simulink model "Multilink_Robot_Arm_control"  (R2019b)
settings: Solver=VariableStepAuto  StartTime=0.0  StopTime=10.0  RelTol=1e-3
libraries: fl_lib x64, fl_ps_legacy_lib x32, nesl_utility x16, simulink x8, ee_lib x8, simulink_extras x4
(part 1 of 2)
settings Model: Creator=Shivanshu  LastModifiedBy=Shivanshu
settings DebuggingCC: SFMachineParentedDataDiag=error

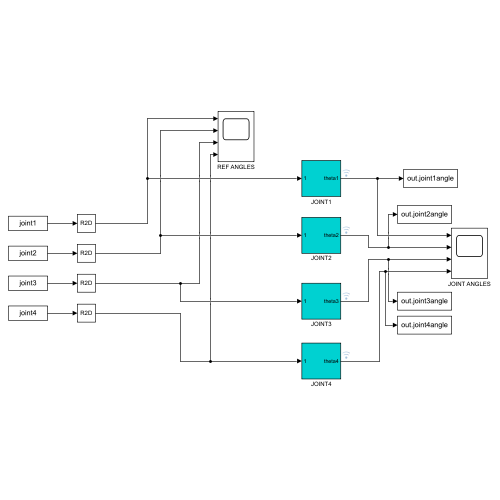
[thumbnail: Simulink's stored preview of the top-level diagram]
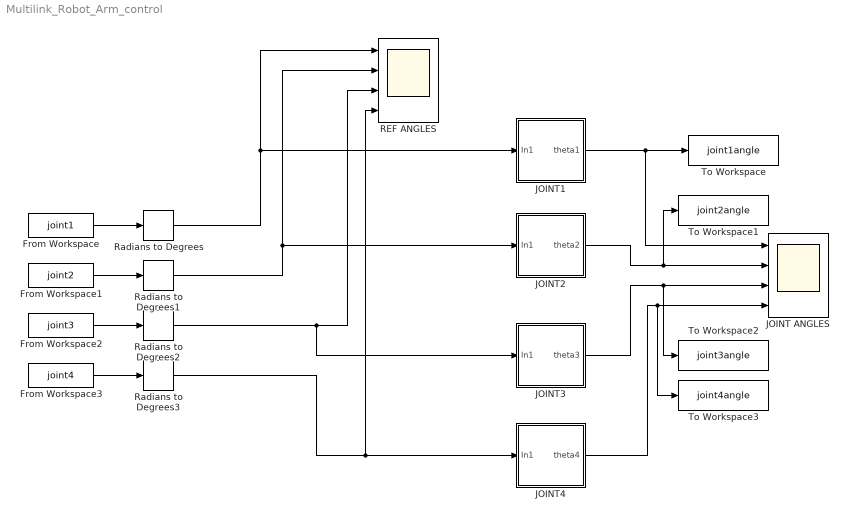
== system Multilink_Robot_Arm_control ==
  From Workspace : FromWorkspace  VariableName=joint1
  From Workspace1 : FromWorkspace  VariableName=joint2
  From Workspace2 : FromWorkspace  VariableName=joint3
  From Workspace3 : FromWorkspace  VariableName=joint4
  JOINT ANGLES : Scope  NumInputPorts=4
  JOINT1 : Subsystem  RequirementInfo={} %GIDa_a5111363_163f_4345_b806_ea7696c3bbc6
  JOINT2 : Subsystem  RequirementInfo={} %GIDa_53c2f0f4_4c39_4c98_aaeb_3fe1813d08cd
  JOINT3 : Subsystem  RequirementInfo={} %GIDa_0e8d513e_7ac6_45e5_95f2_a8ebfc01a2ff
  JOINT4 : Subsystem  RequirementInfo={} %GIDa_b62c3170_0477_431b_a83b_156076afa812
  REF ANGLES : Scope  NumInputPorts=4
  Radians to Degrees{,1..3} (4 alike) : simulink_extras/Transformations/Radians to Degrees
  To Workspace : ToWorkspace  VariableName=joint1angle  SaveFormat=Timeseries  SampleTime=-1
  To Workspace1 : ToWorkspace  VariableName=joint2angle  SaveFormat=Timeseries  SampleTime=-1
  To Workspace2 : ToWorkspace  VariableName=joint3angle  SaveFormat=Timeseries  SampleTime=-1
  To Workspace3 : ToWorkspace  VariableName=joint4angle  SaveFormat=Timeseries  SampleTime=-1
  wires:
  JOINT1/1(theta1) -> To Workspace/1, JOINT ANGLES/1
  JOINT2/1(theta2) -> To Workspace1/1, JOINT ANGLES/2
  JOINT3/1(theta3) -> To Workspace2/1, JOINT ANGLES/3
  JOINT4/1(theta4) -> To Workspace3/1, JOINT ANGLES/4
  From Workspace/1 -> Radians to Degrees/1
  From Workspace1/1 -> Radians to Degrees1/1
  From Workspace2/1 -> Radians to Degrees2/1
  From Workspace3/1 -> Radians to Degrees3/1
  Radians to Degrees/1 -> REF ANGLES/1, JOINT1/1(In1)
  Radians to Degrees1/1 -> REF ANGLES/2, JOINT2/1(In1)
  Radians to Degrees2/1 -> REF ANGLES/3, JOINT3/1(In1)
  Radians to Degrees3/1 -> REF ANGLES/4, JOINT4/1(In1)

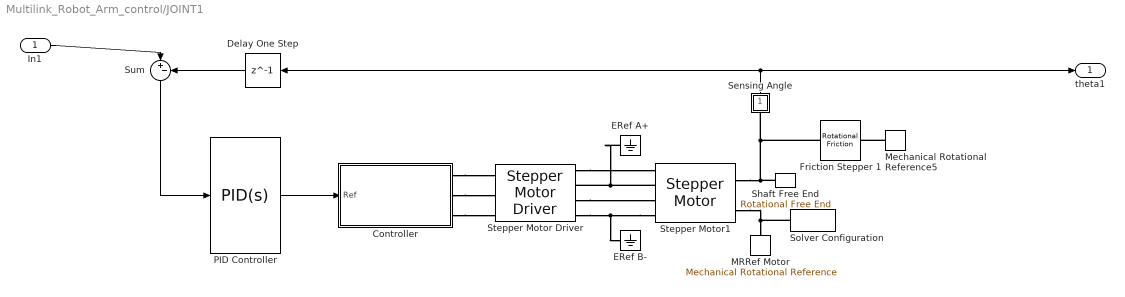
== system Multilink_Robot_Arm_control/JOINT1 ==
  In1 : Inport  RequirementInfo={} %GIDa_bc367b02_467a_4aad_a0ae_789c8a662350
  Controller : Subsystem  RequirementInfo={} %GIDa_f25c4b44_b0be_4777_9ead_d13db3477585  Variant=on  VariantControlMode=label  LabelModeActiveChoice=Speed
      settings: AttributesFormatString=%<BlockChoice>
  Delay One Step : Delay  DelayLength=1
  ERef A+ : fl_lib/Electrical/Electrical Elements/Electrical Reference  RequirementInfo={} %GIDa_75d0a2a4_a7a5_45ce_8433_c1ba340d404c
  ERef B- : fl_lib/Electrical/Electrical Elements/Electrical Reference  RequirementInfo={} %GIDa_a504c1f1_657e_4deb_994a_aa9024733464
  Friction Stepper 1 : fl_lib/Mechanical/Rotational Elements/Rotational Friction  RequirementInfo={} %GIDa_2bd570de_cabd_4835_8246_9ac9ab9b2022  brkwy_trq=3.0e-2 N*m  brkwy_vel=0.03347 rad/s  Col_trq=3.0e-2 N*m  visc_coef=0 N*m/(rad/s)  w_specify=off  w_priority=High  w=0 rad/s  w_nominal_specify=off  w_nominal_unit=rad/s  w_nominal_value=1  t_specify=off  t_priority=High  t=0 N*m  t_nominal_specify=off  t_nominal_unit=N*m  t_nominal_value=1
  MRRef Motor : fl_lib/Mechanical/Rotational Elements/Mechanical Rotational Reference  RequirementInfo={} %GIDa_1e3b9497_35f6_46ed_9d01_e4acec757cd1
  Mechanical Rotational Reference5 : fl_lib/Mechanical/Rotational Elements/Mechanical Rotational Reference  RequirementInfo={} %GIDa_bc527d00_b1b0_4171_a2f1_5d5565209248
  PID Controller : simulink/Continuous/PID Controller  Controller=PID  Form=Parallel  TimeDomain=Continuous-time  SampleTime=-1  IntegratorMethod=Forward Euler  FilterMethod=Forward Euler  ControllerParametersSource=internal  P=6  I=6  D=0  UseFilter=on  N=100  TunerSelectOption=Transfer Function Based (PID Tuner App)  InitialConditionSource=internal  InitialConditionForIntegrator=0  InitialConditionForFilter=0  DifferentiatorICPrevScaledInput=0  ExternalReset=none  TrackingMode=off  Kt=1  LimitOutput=off  UpperSaturationLimit=inf  LowerSaturationLimit=-inf  LinearizeAsGain=on  AntiWindupMode=none  Kb=1  POutMin=[]  POutMax=[]  IOutMin=[]  IOutMax=[]  DOutMin=[]  DOutMax=[]  NOutMin=[]  NOutMax=[]  SumOutMin=[]  SumOutMax=[]  SaturationOutMin=[]  SaturationOutMax=[]  PParamMin=[]  PParamMax=[]  IParamMin=[]  IParamMax=[]  DParamMin=[]  DParamMax=[]  NParamMin=[]  NParamMax=[]  KbParamMin=[]  KbParamMax=[]  KtParamMin=[]  KtParamMax=[]  KbOutMin=[]  KbOutMax=[]  KtOutMin=[]  KtOutMax=[]  IntegratorOutMin=[]  IntegratorOutMax=[]  FilterOutMin=[]  FilterOutMax=[]  SumI1OutMin=[]  SumI1OutMax=[]  SumI2OutMin=[]  SumI2OutMax=[]  SumI3OutMin=[]  SumI3OutMax=[]  SumI4OutMin=[]  SumI4OutMax=[]  SumDOutMin=[]  SumDOutMax=[]  DifferentiatorOutMin=[]  DifferentiatorOutMax=[]  FilterDiffOutCoefMin=[]  FilterDiffOutCoefMax=[]  ReciprocalOutMin=[]  ReciprocalOutMax=[]  SumDenOutMin=[]  SumDenOutMax=[]  SumNumOutMin=[]  SumNumOutMax=[]  DivideOutMin=[]  DivideOutMax=[]  IntegratorContinuousStateAttributes=''  IntegratorStateMustResolveToSignalObject=off  IntegratorRTWStateStorageClass=Auto  FilterContinuousStateAttributes=''  FilterStateMustResolveToSignalObject=off  FilterRTWStateStorageClass=Auto  ParallelPVariant=InternalParameters  IdealPVariant=Disabled  IVariant=InternalParameters  DVariant=InternalParameters  IntegratorVariant=Continuous  SatVariant=Disabled  AWVariant=Passthrough  PCopyVariant=Disabled  TRVariant=Disabled  FdbkBlocksVariant=Forward  IdealPFdbkVariant=Disabled  SatFdbkVariant=Disabled  DerivativeFilterVariant=ContFilter  NVariant=InternalParameters  NCopyVariant=Disabled  FilterICVariant=InternalICsFilter  IntegratorICVariant=InternalICs  ExternalResetVariant=Disabled  TRSumVariant=Passthrough  SumFdbkVariant=Disabled  SumVariant=Sum_PID
  Sensing Angle : Subsystem  RequirementInfo={} %GIDa_61ee900a_055d_4dbe_8670_1389978465cb
      mask Display: disp('a')
  Shaft Free End : fl_lib/Mechanical/Rotational Elements/Rotational Free End  RequirementInfo={} %GIDa_07e10779_510a_43cf_bd47_0467719cabe3  w_specify=off  w_priority=None  w=0 rad/s  w_nominal_specify=off  w_nominal_unit=rad/s  w_nominal_value=1
      settings: SourceProductBaseCode=SS
  Solver Configuration : nesl_utility/Solver Configuration  RequirementInfo={} %GIDa_25e696ba_71a2_4de9_b9eb_ebb28de57fd1  PhysicalDomain=network_engine_domain  SubClassName=solver  LeftPortType=input  RightPortType=generic  Tones=[]  Harmonics=[]  SimulateNoise=off  Profile=off  UseLocalSampling=off  EnableSwitchedLinearOptims=on  FrequencyDomain=off  UseCCode=off  RelTol=0.001  AbsTol=1e-06  MinStep=1e-09  ToWorkspace=off  RevertToSquareIcSolve=off  NumHomotopyIterations=100  PhasorMode=off  PhasorModeNumHarmonics=1  DoDC=off  ResidualTolerance=1e-9  UseLocalSolver=off  LocalSolverChoice=NE_BACKWARD_EULER_ADVANCER  LocalSolverSampleTime=.001  DoFixedCost=off  MaxNonlinIter=3  MaxModeIter=2  ComputeImpulses=off  ImpulseIterations=2  LinearAlgebra=auto  EquationFormulation=NE_TIME_EF  DelaysMemoryBudget=1024  AutomaticFiltering=on  FilteringTimeConstant=0.001  PartitionStorageMethod=AS_NEEDED  PartitionMemoryBudget=1024  PartitionMethod=FAST
      settings: SourceProductBaseCode=PW,SS
  Stepper Motor Driver : ee_lib/Electromechanical/Reluctance & Stepper/Stepper Motor Driver  RequirementInfo={} %GIDa_6add52ff_d6dc_4229_b9b5_c0a05064c9a5  step_or_av=ee.enum.electromech.simulationMode.stepping  step_rate_per_volt=10 Hz/V  Venable=2.5 V  Vreverse=2.5 V  supply_ports=ee.enum.supply_ports.hidesupply  Vm=5 V  Vsupply=10 V  half_stepping=ee.enum.electromech.steppingModeAveraged.fullStep  stepping_mode=ee.enum.electromech.steppingMode.microStep  numMicroSteps=4  Im=1.2 A
      settings: SourceProductBaseCode=PS  InternalSimscapePortConfiguration="{\"Bottom\":[],\"Left\":[{\"id\":\"ENA\",\"label\":\"ENA\",\"type\":\"foundation.electrical.electrical\"},{\"id\":\"REF\",\"label\":\"REF\",\"type\":\"foundation.electrical.electrical\"},{\"id\":\"REV\",\"label\":\"REV\",\"type\":\"foundation.electrical.electrical\"}],\"Right\":[{\"id\":\"pA\",\"label\":\"A+\",\"type\":\"foundation.electrical.electrical\"},{\"id\":\"nA\",\"label\":\"A-\",\"type\":\"foundation.electrical.electrical\"},{\"id\":\"pB\",\"label\":\"B+\",\"type\":\"foundation.electrical.electrical\"},{\"id\":\"nB\",\"label\":\"B-\",\"type\":\"foundation.electrical.electrical\"}],\"Top\":[]}"
  Stepper Motor1 : ee_lib/Electromechanical/Reluctance & Stepper/Stepper Motor  RequirementInfo={} %GIDa_899a14fe_f658_4fbd_8da8_089dcdef886b  step_or_av=1  Ra=0.55 Ohm  La=0.0015 H  Km=0.19 N*m/A  Td=0 N*m  Rm=Inf Ohm  w_vec=[ 0 1000 3e+3 ] rpm  T_vec=[ 2 2 1 ] N*m  assert_if_slipping=0  J_total=1e-4 kg*m^2  max_step_rate=10 Hz  Step=1.8 deg  J=4.5e-05 kg*m^2  B=1e-02 N*m/(rad/s)  speed0=0 rpm  theta0=0 deg  alpha=[.00393, .00393] 1/K  Tmeas=25 degC  Tmeas2=125 degC  T_vec2=[1.7, 1.7, .85] N*m  half_stepping=ee.enum.electromech.steppingModeAveraged.fullStep  thermal_masses=[100, 100] J/K  initial_temperatures=[25, 25] degC  rotor_thermal_mass=50 J/K  rotor_initial_temperature=25 degC  Rm_percent_rotor=90
      settings: SourceProductBaseCode=PS  InternalSimscapePortConfiguration="{\"Bottom\":[],\"Left\":[{\"id\":\"pA\",\"label\":\"A+\",\"type\":\"foundation.electrical.electrical\"},{\"id\":\"nA\",\"label\":\"A-\",\"type\":\"foundation.electrical.electrical\"},{\"id\":\"pB\",\"label\":\"B+\",\"type\":\"foundation.electrical.electrical\"},{\"id\":\"nB\",\"label\":\"B-\",\"type\":\"foundation.electrical.electrical\"}],\"Right\":[{\"id\":\"R\",\"label\":\"R\",\"type\":\"foundation.mechanical.rotational.rotational\"},{\"id\":\"C\",\"label\":\"C\",\"type\":\"foundation.mechanical.rotational.rotational\"}],\"Top\":[]}"
  Sum : Sum  RequirementInfo={} %GIDa_b6fd566b_487f_4eb7_8ec1_d8d119f2a8ee  Inputs=|+-
  theta1 : Outport  RequirementInfo={} %GIDa_3b18913c_887e_46dc_8d95_ea9fed50315c
  wires:
  In1/1 -> Sum/1
  Sum/1 -> PID Controller/1
  Sensing Angle/1(theta) -> Delay One Step/1, theta1/1
  PID Controller/1 -> Controller/1(Ref)
  Delay One Step/1 -> Sum/2
  connections:
  Controller/RConn2 -- Stepper Motor Driver/LConn2
  Stepper Motor Driver/RConn1 -- Stepper Motor1/LConn1
  Controller/RConn1 -- Stepper Motor Driver/LConn1
  Solver Configuration/RConn1 -- Stepper Motor1/RConn2 -- MRRef Motor/LConn1
  ERef A+/LConn1 -- Stepper Motor1/LConn2 -- Stepper Motor Driver/RConn2
  Stepper Motor Driver/RConn3 -- Stepper Motor1/LConn3
  Mechanical Rotational Reference5/LConn1 -- Friction Stepper 1/RConn1
  Controller/RConn3 -- Stepper Motor Driver/LConn3
  Stepper Motor1/LConn4 -- Stepper Motor Driver/RConn4 -- ERef B-/LConn1
  Sensing Angle/LConn1 -- Friction Stepper 1/LConn1 -- Shaft Free End/LConn1 -- Stepper Motor1/RConn1

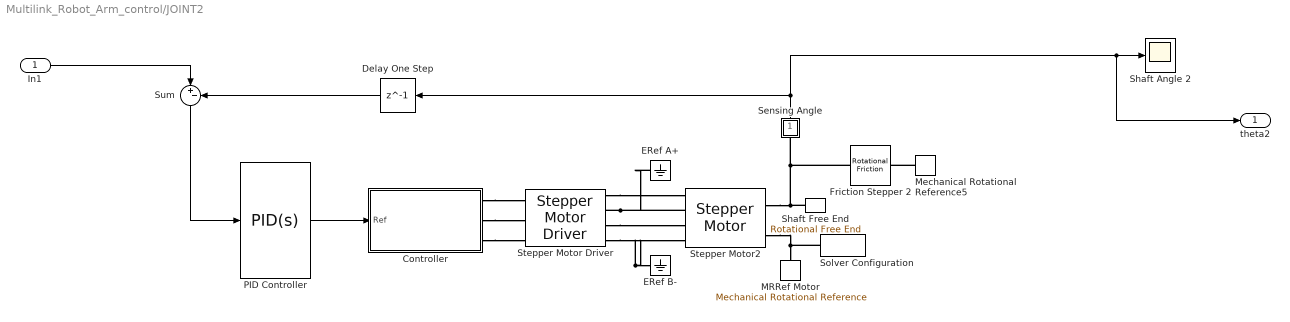
== system Multilink_Robot_Arm_control/JOINT2 ==
  In1 : Inport  RequirementInfo={} %GIDa_f4ca45d3_978e_4626_b159_1459f1220710
  Controller : Subsystem  RequirementInfo={} %GIDa_6b7040c3_f640_4a87_bf66_e8c964445a67  Variant=on  VariantControlMode=label  LabelModeActiveChoice=Speed
      settings: AttributesFormatString=%<BlockChoice>
  Delay One Step : Delay  DelayLength=1
  ERef A+ : fl_lib/Electrical/Electrical Elements/Electrical Reference  RequirementInfo={} %GIDa_7d701a76_5455_4d0b_9fe6_36236dcac0c6
  ERef B- : fl_lib/Electrical/Electrical Elements/Electrical Reference  RequirementInfo={} %GIDa_2b6e6a9c_19e8_479a_8975_04df8b082307
  Friction Stepper 2 : fl_lib/Mechanical/Rotational Elements/Rotational Friction  RequirementInfo={} %GIDa_3b81cbd5_c7e2_440a_aa27_f55ca4e17504  brkwy_trq=3.0e-2 N*m  brkwy_vel=0.03347 rad/s  Col_trq=3.0e-2 N*m  visc_coef=0 N*m/(rad/s)  w_specify=off  w_priority=High  w=0 rad/s  w_nominal_specify=off  w_nominal_unit=rad/s  w_nominal_value=1  t_specify=off  t_priority=High  t=0 N*m  t_nominal_specify=off  t_nominal_unit=N*m  t_nominal_value=1
  MRRef Motor : fl_lib/Mechanical/Rotational Elements/Mechanical Rotational Reference  RequirementInfo={} %GIDa_51d91c63_f685_4d63_85ad_6bfab74a6a61
  Mechanical Rotational Reference5 : fl_lib/Mechanical/Rotational Elements/Mechanical Rotational Reference  RequirementInfo={} %GIDa_2f9bb432_5c38_4f9c_b804_5817bac98aae
  PID Controller : simulink/Continuous/PID Controller  Controller=PID  Form=Parallel  TimeDomain=Continuous-time  SampleTime=-1  IntegratorMethod=Forward Euler  FilterMethod=Forward Euler  ControllerParametersSource=internal  P=6  I=6  D=0  UseFilter=on  N=100  TunerSelectOption=Transfer Function Based (PID Tuner App)  InitialConditionSource=internal  InitialConditionForIntegrator=0  InitialConditionForFilter=0  DifferentiatorICPrevScaledInput=0  ExternalReset=none  TrackingMode=off  Kt=1  LimitOutput=off  UpperSaturationLimit=inf  LowerSaturationLimit=-inf  LinearizeAsGain=on  AntiWindupMode=none  Kb=1  POutMin=[]  POutMax=[]  IOutMin=[]  IOutMax=[]  DOutMin=[]  DOutMax=[]  NOutMin=[]  NOutMax=[]  SumOutMin=[]  SumOutMax=[]  SaturationOutMin=[]  SaturationOutMax=[]  PParamMin=[]  PParamMax=[]  IParamMin=[]  IParamMax=[]  DParamMin=[]  DParamMax=[]  NParamMin=[]  NParamMax=[]  KbParamMin=[]  KbParamMax=[]  KtParamMin=[]  KtParamMax=[]  KbOutMin=[]  KbOutMax=[]  KtOutMin=[]  KtOutMax=[]  IntegratorOutMin=[]  IntegratorOutMax=[]  FilterOutMin=[]  FilterOutMax=[]  SumI1OutMin=[]  SumI1OutMax=[]  SumI2OutMin=[]  SumI2OutMax=[]  SumI3OutMin=[]  SumI3OutMax=[]  SumI4OutMin=[]  SumI4OutMax=[]  SumDOutMin=[]  SumDOutMax=[]  DifferentiatorOutMin=[]  DifferentiatorOutMax=[]  FilterDiffOutCoefMin=[]  FilterDiffOutCoefMax=[]  ReciprocalOutMin=[]  ReciprocalOutMax=[]  SumDenOutMin=[]  SumDenOutMax=[]  SumNumOutMin=[]  SumNumOutMax=[]  DivideOutMin=[]  DivideOutMax=[]  IntegratorContinuousStateAttributes=''  IntegratorStateMustResolveToSignalObject=off  IntegratorRTWStateStorageClass=Auto  FilterContinuousStateAttributes=''  FilterStateMustResolveToSignalObject=off  FilterRTWStateStorageClass=Auto  ParallelPVariant=InternalParameters  IdealPVariant=Disabled  IVariant=InternalParameters  DVariant=InternalParameters  IntegratorVariant=Continuous  SatVariant=Disabled  AWVariant=Passthrough  PCopyVariant=Disabled  TRVariant=Disabled  FdbkBlocksVariant=Forward  IdealPFdbkVariant=Disabled  SatFdbkVariant=Disabled  DerivativeFilterVariant=ContFilter  NVariant=InternalParameters  NCopyVariant=Disabled  FilterICVariant=InternalICsFilter  IntegratorICVariant=InternalICs  ExternalResetVariant=Disabled  TRSumVariant=Passthrough  SumFdbkVariant=Disabled  SumVariant=Sum_PID
  Sensing Angle : Subsystem  RequirementInfo={} %GIDa_232d717f_c322_40c5_b89a_c1b1251fbd93
      mask Display: disp('a')
  Shaft Angle 2 : Scope
      settings: RequirementInfo={} %GIDa_297c8822_2cda_45b9_9bbf_834b808f164e
  Shaft Free End : fl_lib/Mechanical/Rotational Elements/Rotational Free End  RequirementInfo={} %GIDa_37b8bc85_4a06_41f7_9255_d1690db4786c  w_specify=off  w_priority=None  w=0 rad/s  w_nominal_specify=off  w_nominal_unit=rad/s  w_nominal_value=1
      settings: SourceProductBaseCode=SS
  Solver Configuration : nesl_utility/Solver Configuration  RequirementInfo={} %GIDa_0cce2d2f_311b_4f52_8ef3_4f9435f396f5  PhysicalDomain=network_engine_domain  SubClassName=solver  LeftPortType=input  RightPortType=generic  Tones=[]  Harmonics=[]  SimulateNoise=off  Profile=off  UseLocalSampling=off  EnableSwitchedLinearOptims=on  FrequencyDomain=off  UseCCode=off  RelTol=0.001  AbsTol=1e-06  MinStep=1e-09  ToWorkspace=off  RevertToSquareIcSolve=off  NumHomotopyIterations=100  PhasorMode=off  PhasorModeNumHarmonics=1  DoDC=off  ResidualTolerance=1e-9  UseLocalSolver=off  LocalSolverChoice=NE_BACKWARD_EULER_ADVANCER  LocalSolverSampleTime=.001  DoFixedCost=off  MaxNonlinIter=3  MaxModeIter=2  ComputeImpulses=off  ImpulseIterations=2  LinearAlgebra=auto  EquationFormulation=NE_TIME_EF  DelaysMemoryBudget=1024  AutomaticFiltering=on  FilteringTimeConstant=0.001  PartitionStorageMethod=AS_NEEDED  PartitionMemoryBudget=1024  PartitionMethod=FAST
      settings: SourceProductBaseCode=PW,SS
  Stepper Motor Driver : ee_lib/Electromechanical/Reluctance & Stepper/Stepper Motor Driver  RequirementInfo={} %GIDa_fcbdaa05_6c4a_4a4c_aad1_4b4ef2482798  step_or_av=ee.enum.electromech.simulationMode.stepping  step_rate_per_volt=10 Hz/V  Venable=2.5 V  Vreverse=2.5 V  supply_ports=ee.enum.supply_ports.hidesupply  Vm=5 V  Vsupply=10 V  half_stepping=ee.enum.electromech.steppingModeAveraged.fullStep  stepping_mode=ee.enum.electromech.steppingMode.microStep  numMicroSteps=4  Im=1.2 A
      settings: SourceProductBaseCode=PS  InternalSimscapePortConfiguration="{\"Bottom\":[],\"Left\":[{\"id\":\"ENA\",\"label\":\"ENA\",\"type\":\"foundation.electrical.electrical\"},{\"id\":\"REF\",\"label\":\"REF\",\"type\":\"foundation.electrical.electrical\"},{\"id\":\"REV\",\"label\":\"REV\",\"type\":\"foundation.electrical.electrical\"}],\"Right\":[{\"id\":\"pA\",\"label\":\"A+\",\"type\":\"foundation.electrical.electrical\"},{\"id\":\"nA\",\"label\":\"A-\",\"type\":\"foundation.electrical.electrical\"},{\"id\":\"pB\",\"label\":\"B+\",\"type\":\"foundation.electrical.electrical\"},{\"id\":\"nB\",\"label\":\"B-\",\"type\":\"foundation.electrical.electrical\"}],\"Top\":[]}"
  Stepper Motor2 : ee_lib/Electromechanical/Reluctance & Stepper/Stepper Motor  RequirementInfo={} %GIDa_5d4e60a0_db2c_4cac_ba81_88f1c1856eb7  step_or_av=1  Ra=0.55 Ohm  La=0.0015 H  Km=0.19 N*m/A  Td=0 N*m  Rm=Inf Ohm  w_vec=[ 0 1000 3e+3 ] rpm  T_vec=[ 2 2 1 ] N*m  assert_if_slipping=0  J_total=1e-4 kg*m^2  max_step_rate=10 Hz  Step=1.8 deg  J=4.5e-05 kg*m^2  B=1e-02 N*m/(rad/s)  speed0=0 rpm  theta0=0 deg  alpha=[.00393, .00393] 1/K  Tmeas=25 degC  Tmeas2=125 degC  T_vec2=[1.7, 1.7, .85] N*m  half_stepping=ee.enum.electromech.steppingModeAveraged.fullStep  thermal_masses=[100, 100] J/K  initial_temperatures=[25, 25] degC  rotor_thermal_mass=50 J/K  rotor_initial_temperature=25 degC  Rm_percent_rotor=90
      settings: SourceProductBaseCode=PS  InternalSimscapePortConfiguration="{\"Bottom\":[],\"Left\":[{\"id\":\"pA\",\"label\":\"A+\",\"type\":\"foundation.electrical.electrical\"},{\"id\":\"nA\",\"label\":\"A-\",\"type\":\"foundation.electrical.electrical\"},{\"id\":\"pB\",\"label\":\"B+\",\"type\":\"foundation.electrical.electrical\"},{\"id\":\"nB\",\"label\":\"B-\",\"type\":\"foundation.electrical.electrical\"}],\"Right\":[{\"id\":\"R\",\"label\":\"R\",\"type\":\"foundation.mechanical.rotational.rotational\"},{\"id\":\"C\",\"label\":\"C\",\"type\":\"foundation.mechanical.rotational.rotational\"}],\"Top\":[]}"
  Sum : Sum  RequirementInfo={} %GIDa_b6aee27b_9591_4b6c_ad0b_9133f92eb5c4  Inputs=|+-
  theta2 : Outport  RequirementInfo={} %GIDa_8e4d7c24_2bc4_4b58_bd58_441e199132e9
  wires:
  PID Controller/1 -> Controller/1(Ref)
  Sensing Angle/1(theta) -> Delay One Step/1, theta2/1, Shaft Angle 2/1
  Sum/1 -> PID Controller/1
  In1/1 -> Sum/1
  Delay One Step/1 -> Sum/2
  connections:
  Stepper Motor2/RConn1 -- Shaft Free End/LConn1 -- Friction Stepper 2/LConn1 -- Sensing Angle/LConn1
  ERef B-/LConn1 -- Stepper Motor Driver/RConn4 -- Stepper Motor2/LConn4
  Controller/RConn3 -- Stepper Motor Driver/LConn3
  Mechanical Rotational Reference5/LConn1 -- Friction Stepper 2/RConn1
  Stepper Motor Driver/RConn3 -- Stepper Motor2/LConn3
  Stepper Motor Driver/RConn2 -- Stepper Motor2/LConn2 -- ERef A+/LConn1
  MRRef Motor/LConn1 -- Stepper Motor2/RConn2 -- Solver Configuration/RConn1
  Controller/RConn1 -- Stepper Motor Driver/LConn1
  Stepper Motor Driver/RConn1 -- Stepper Motor2/LConn1
  Controller/RConn2 -- Stepper Motor Driver/LConn2

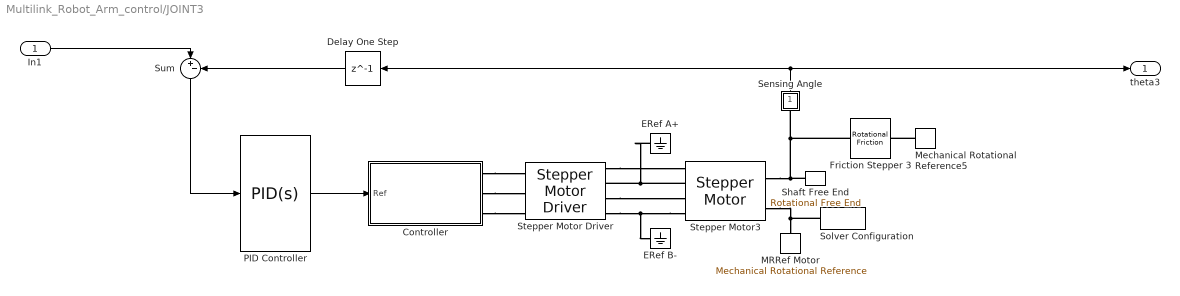
== system Multilink_Robot_Arm_control/JOINT3 ==
  In1 : Inport  RequirementInfo={} %GIDa_28432bb8_aa37_4d4e_b110_403d32239de1
  Controller : Subsystem  RequirementInfo={} %GIDa_5d478c58_e3fd_4507_a31d_2d3ccaac3dcf  Variant=on  VariantControlMode=label  LabelModeActiveChoice=Speed
      settings: AttributesFormatString=%<BlockChoice>
  Delay One Step : Delay  DelayLength=1
  ERef A+ : fl_lib/Electrical/Electrical Elements/Electrical Reference  RequirementInfo={} %GIDa_d73b157d_238c_453f_8c17_4358983f74fe
  ERef B- : fl_lib/Electrical/Electrical Elements/Electrical Reference  RequirementInfo={} %GIDa_32ef3304_c487_42ce_93ff_e20cd95a236c
  Friction Stepper 3 : fl_lib/Mechanical/Rotational Elements/Rotational Friction  RequirementInfo={} %GIDa_ecb45a01_979d_4b61_915c_a4ed1185d199  brkwy_trq=3.0e-2 N*m  brkwy_vel=0.03347 rad/s  Col_trq=3.0e-2 N*m  visc_coef=0 N*m/(rad/s)  w_specify=off  w_priority=High  w=0 rad/s  w_nominal_specify=off  w_nominal_unit=rad/s  w_nominal_value=1  t_specify=off  t_priority=High  t=0 N*m  t_nominal_specify=off  t_nominal_unit=N*m  t_nominal_value=1
  MRRef Motor : fl_lib/Mechanical/Rotational Elements/Mechanical Rotational Reference  RequirementInfo={} %GIDa_d56416ed_b9cf_4024_bb29_94cb1fca91c8
  Mechanical Rotational Reference5 : fl_lib/Mechanical/Rotational Elements/Mechanical Rotational Reference  RequirementInfo={} %GIDa_4cc99843_da0e_4d37_b35a_a3b83fd20b21
  PID Controller : simulink/Continuous/PID Controller  Controller=PID  Form=Parallel  TimeDomain=Continuous-time  SampleTime=-1  IntegratorMethod=Forward Euler  FilterMethod=Forward Euler  ControllerParametersSource=internal  P=6  I=6  D=0  UseFilter=on  N=100  TunerSelectOption=Transfer Function Based (PID Tuner App)  InitialConditionSource=internal  InitialConditionForIntegrator=0  InitialConditionForFilter=0  DifferentiatorICPrevScaledInput=0  ExternalReset=none  TrackingMode=off  Kt=1  LimitOutput=off  UpperSaturationLimit=inf  LowerSaturationLimit=-inf  LinearizeAsGain=on  AntiWindupMode=none  Kb=1  POutMin=[]  POutMax=[]  IOutMin=[]  IOutMax=[]  DOutMin=[]  DOutMax=[]  NOutMin=[]  NOutMax=[]  SumOutMin=[]  SumOutMax=[]  SaturationOutMin=[]  SaturationOutMax=[]  PParamMin=[]  PParamMax=[]  IParamMin=[]  IParamMax=[]  DParamMin=[]  DParamMax=[]  NParamMin=[]  NParamMax=[]  KbParamMin=[]  KbParamMax=[]  KtParamMin=[]  KtParamMax=[]  KbOutMin=[]  KbOutMax=[]  KtOutMin=[]  KtOutMax=[]  IntegratorOutMin=[]  IntegratorOutMax=[]  FilterOutMin=[]  FilterOutMax=[]  SumI1OutMin=[]  SumI1OutMax=[]  SumI2OutMin=[]  SumI2OutMax=[]  SumI3OutMin=[]  SumI3OutMax=[]  SumI4OutMin=[]  SumI4OutMax=[]  SumDOutMin=[]  SumDOutMax=[]  DifferentiatorOutMin=[]  DifferentiatorOutMax=[]  FilterDiffOutCoefMin=[]  FilterDiffOutCoefMax=[]  ReciprocalOutMin=[]  ReciprocalOutMax=[]  SumDenOutMin=[]  SumDenOutMax=[]  SumNumOutMin=[]  SumNumOutMax=[]  DivideOutMin=[]  DivideOutMax=[]  IntegratorContinuousStateAttributes=''  IntegratorStateMustResolveToSignalObject=off  IntegratorRTWStateStorageClass=Auto  FilterContinuousStateAttributes=''  FilterStateMustResolveToSignalObject=off  FilterRTWStateStorageClass=Auto  ParallelPVariant=InternalParameters  IdealPVariant=Disabled  IVariant=InternalParameters  DVariant=InternalParameters  IntegratorVariant=Continuous  SatVariant=Disabled  AWVariant=Passthrough  PCopyVariant=Disabled  TRVariant=Disabled  FdbkBlocksVariant=Forward  IdealPFdbkVariant=Disabled  SatFdbkVariant=Disabled  DerivativeFilterVariant=ContFilter  NVariant=InternalParameters  NCopyVariant=Disabled  FilterICVariant=InternalICsFilter  IntegratorICVariant=InternalICs  ExternalResetVariant=Disabled  TRSumVariant=Passthrough  SumFdbkVariant=Disabled  SumVariant=Sum_PID
  Sensing Angle : Subsystem  RequirementInfo={} %GIDa_d82698ec_e094_4b3b_bbcf_2493d5f96c19
      mask Display: disp('a')
  Shaft Free End : fl_lib/Mechanical/Rotational Elements/Rotational Free End  RequirementInfo={} %GIDa_b70c04a6_8619_4adb_b6bd_7b6e45112bf0  w_specify=off  w_priority=None  w=0 rad/s  w_nominal_specify=off  w_nominal_unit=rad/s  w_nominal_value=1
      settings: SourceProductBaseCode=SS
  Solver Configuration : nesl_utility/Solver Configuration  RequirementInfo={} %GIDa_ddeb65e0_6989_4173_8d23_6178a1407ca8  PhysicalDomain=network_engine_domain  SubClassName=solver  LeftPortType=input  RightPortType=generic  Tones=[]  Harmonics=[]  SimulateNoise=off  Profile=off  UseLocalSampling=off  EnableSwitchedLinearOptims=on  FrequencyDomain=off  UseCCode=off  RelTol=0.001  AbsTol=1e-06  MinStep=1e-09  ToWorkspace=off  RevertToSquareIcSolve=off  NumHomotopyIterations=100  PhasorMode=off  PhasorModeNumHarmonics=1  DoDC=off  ResidualTolerance=1e-9  UseLocalSolver=off  LocalSolverChoice=NE_BACKWARD_EULER_ADVANCER  LocalSolverSampleTime=.001  DoFixedCost=off  MaxNonlinIter=3  MaxModeIter=2  ComputeImpulses=off  ImpulseIterations=2  LinearAlgebra=auto  EquationFormulation=NE_TIME_EF  DelaysMemoryBudget=1024  AutomaticFiltering=on  FilteringTimeConstant=0.001  PartitionStorageMethod=AS_NEEDED  PartitionMemoryBudget=1024  PartitionMethod=FAST
      settings: SourceProductBaseCode=PW,SS
  Stepper Motor Driver : ee_lib/Electromechanical/Reluctance & Stepper/Stepper Motor Driver  RequirementInfo={} %GIDa_999a8bc2_e412_4702_ab2c_f62fbccdaa56  step_or_av=ee.enum.electromech.simulationMode.stepping  step_rate_per_volt=10 Hz/V  Venable=2.5 V  Vreverse=2.5 V  supply_ports=ee.enum.supply_ports.hidesupply  Vm=5 V  Vsupply=10 V  half_stepping=ee.enum.electromech.steppingModeAveraged.fullStep  stepping_mode=ee.enum.electromech.steppingMode.microStep  numMicroSteps=4  Im=1.2 A
      settings: SourceProductBaseCode=PS  InternalSimscapePortConfiguration="{\"Bottom\":[],\"Left\":[{\"id\":\"ENA\",\"label\":\"ENA\",\"type\":\"foundation.electrical.electrical\"},{\"id\":\"REF\",\"label\":\"REF\",\"type\":\"foundation.electrical.electrical\"},{\"id\":\"REV\",\"label\":\"REV\",\"type\":\"foundation.electrical.electrical\"}],\"Right\":[{\"id\":\"pA\",\"label\":\"A+\",\"type\":\"foundation.electrical.electrical\"},{\"id\":\"nA\",\"label\":\"A-\",\"type\":\"foundation.electrical.electrical\"},{\"id\":\"pB\",\"label\":\"B+\",\"type\":\"foundation.electrical.electrical\"},{\"id\":\"nB\",\"label\":\"B-\",\"type\":\"foundation.electrical.electrical\"}],\"Top\":[]}"
  Stepper Motor3 : ee_lib/Electromechanical/Reluctance & Stepper/Stepper Motor  RequirementInfo={} %GIDa_276add06_ab0f_4deb_81ad_d8753f8d1500  step_or_av=1  Ra=0.55 Ohm  La=0.0015 H  Km=0.19 N*m/A  Td=0 N*m  Rm=Inf Ohm  w_vec=[ 0 1000 3e+3 ] rpm  T_vec=[ 2 2 1 ] N*m  assert_if_slipping=0  J_total=1e-4 kg*m^2  max_step_rate=10 Hz  Step=1.8 deg  J=4.5e-05 kg*m^2  B=1e-02 N*m/(rad/s)  speed0=0 rpm  theta0=0 deg  alpha=[.00393, .00393] 1/K  Tmeas=25 degC  Tmeas2=125 degC  T_vec2=[1.7, 1.7, .85] N*m  half_stepping=ee.enum.electromech.steppingModeAveraged.fullStep  thermal_masses=[100, 100] J/K  initial_temperatures=[25, 25] degC  rotor_thermal_mass=50 J/K  rotor_initial_temperature=25 degC  Rm_percent_rotor=90
      settings: SourceProductBaseCode=PS  InternalSimscapePortConfiguration="{\"Bottom\":[],\"Left\":[{\"id\":\"pA\",\"label\":\"A+\",\"type\":\"foundation.electrical.electrical\"},{\"id\":\"nA\",\"label\":\"A-\",\"type\":\"foundation.electrical.electrical\"},{\"id\":\"pB\",\"label\":\"B+\",\"type\":\"foundation.electrical.electrical\"},{\"id\":\"nB\",\"label\":\"B-\",\"type\":\"foundation.electrical.electrical\"}],\"Right\":[{\"id\":\"R\",\"label\":\"R\",\"type\":\"foundation.mechanical.rotational.rotational\"},{\"id\":\"C\",\"label\":\"C\",\"type\":\"foundation.mechanical.rotational.rotational\"}],\"Top\":[]}"
  Sum : Sum  RequirementInfo={} %GIDa_8e07d75a_f78d_4ebf_806b_f1de4b24253f  Inputs=|+-
  theta3 : Outport  RequirementInfo={} %GIDa_5111fc7a_9fbb_4b0a_b4ad_cea7d8288aa3
  wires:
  In1/1 -> Sum/1
  Sum/1 -> PID Controller/1
  Sensing Angle/1(theta) -> theta3/1, Delay One Step/1
  PID Controller/1 -> Controller/1(Ref)
  Delay One Step/1 -> Sum/2
  connections:
  Controller/RConn2 -- Stepper Motor Driver/LConn2
  Stepper Motor Driver/RConn1 -- Stepper Motor3/LConn1
  Controller/RConn1 -- Stepper Motor Driver/LConn1
  Solver Configuration/RConn1 -- Stepper Motor3/RConn2 -- MRRef Motor/LConn1
  ERef A+/LConn1 -- Stepper Motor3/LConn2 -- Stepper Motor Driver/RConn2
  Stepper Motor Driver/RConn3 -- Stepper Motor3/LConn3
  Mechanical Rotational Reference5/LConn1 -- Friction Stepper 3/RConn1
  Controller/RConn3 -- Stepper Motor Driver/LConn3
  Stepper Motor3/LConn4 -- Stepper Motor Driver/RConn4 -- ERef B-/LConn1
  Sensing Angle/LConn1 -- Friction Stepper 3/LConn1 -- Shaft Free End/LConn1 -- Stepper Motor3/RConn1

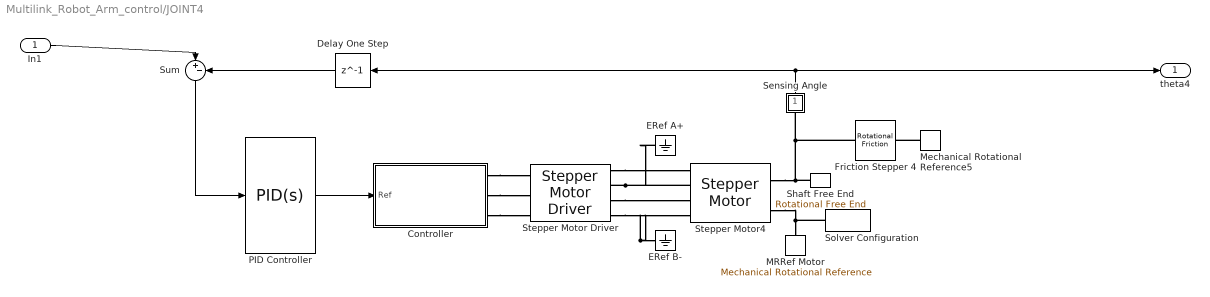
== system Multilink_Robot_Arm_control/JOINT4 ==
  In1 : Inport  RequirementInfo={} %GIDa_a25105c6_d545_4b1e_8372_0194c094cd3e
  Controller : Subsystem  RequirementInfo={} %GIDa_e809cee0_85a3_4087_9478_f055bcae0bb6  Variant=on  VariantControlMode=label  LabelModeActiveChoice=Speed
      settings: AttributesFormatString=%<BlockChoice>
  Delay One Step : Delay  DelayLength=1
  ERef A+ : fl_lib/Electrical/Electrical Elements/Electrical Reference  RequirementInfo={} %GIDa_06e6757e_361c_4bf2_9cda_edb931ec7425
  ERef B- : fl_lib/Electrical/Electrical Elements/Electrical Reference  RequirementInfo={} %GIDa_c9076a18_acbc_418b_9d05_725e6e0abcb5
  Friction Stepper 4 : fl_lib/Mechanical/Rotational Elements/Rotational Friction  RequirementInfo={} %GIDa_63715b5d_3df4_4a2e_9b5d_220454839182  brkwy_trq=3.0e-2 N*m  brkwy_vel=0.03347 rad/s  Col_trq=3.0e-2 N*m  visc_coef=0 N*m/(rad/s)  w_specify=off  w_priority=High  w=0 rad/s  w_nominal_specify=off  w_nominal_unit=rad/s  w_nominal_value=1  t_specify=off  t_priority=High  t=0 N*m  t_nominal_specify=off  t_nominal_unit=N*m  t_nominal_value=1
  MRRef Motor : fl_lib/Mechanical/Rotational Elements/Mechanical Rotational Reference  RequirementInfo={} %GIDa_3a1885fc_cad5_4f2c_9579_3c10e2e35f40
  Mechanical Rotational Reference5 : fl_lib/Mechanical/Rotational Elements/Mechanical Rotational Reference  RequirementInfo={} %GIDa_73654c36_78d0_4a6e_9510_4897320a6c2b
  PID Controller : simulink/Continuous/PID Controller  Controller=PID  Form=Parallel  TimeDomain=Continuous-time  SampleTime=-1  IntegratorMethod=Forward Euler  FilterMethod=Forward Euler  ControllerParametersSource=internal  P=6  I=6  D=0  UseFilter=on  N=100  TunerSelectOption=Transfer Function Based (PID Tuner App)  InitialConditionSource=internal  InitialConditionForIntegrator=0  InitialConditionForFilter=0  DifferentiatorICPrevScaledInput=0  ExternalReset=none  TrackingMode=off  Kt=1  LimitOutput=off  UpperSaturationLimit=inf  LowerSaturationLimit=-inf  LinearizeAsGain=on  AntiWindupMode=none  Kb=1  POutMin=[]  POutMax=[]  IOutMin=[]  IOutMax=[]  DOutMin=[]  DOutMax=[]  NOutMin=[]  NOutMax=[]  SumOutMin=[]  SumOutMax=[]  SaturationOutMin=[]  SaturationOutMax=[]  PParamMin=[]  PParamMax=[]  IParamMin=[]  IParamMax=[]  DParamMin=[]  DParamMax=[]  NParamMin=[]  NParamMax=[]  KbParamMin=[]  KbParamMax=[]  KtParamMin=[]  KtParamMax=[]  KbOutMin=[]  KbOutMax=[]  KtOutMin=[]  KtOutMax=[]  IntegratorOutMin=[]  IntegratorOutMax=[]  FilterOutMin=[]  FilterOutMax=[]  SumI1OutMin=[]  SumI1OutMax=[]  SumI2OutMin=[]  SumI2OutMax=[]  SumI3OutMin=[]  SumI3OutMax=[]  SumI4OutMin=[]  SumI4OutMax=[]  SumDOutMin=[]  SumDOutMax=[]  DifferentiatorOutMin=[]  DifferentiatorOutMax=[]  FilterDiffOutCoefMin=[]  FilterDiffOutCoefMax=[]  ReciprocalOutMin=[]  ReciprocalOutMax=[]  SumDenOutMin=[]  SumDenOutMax=[]  SumNumOutMin=[]  SumNumOutMax=[]  DivideOutMin=[]  DivideOutMax=[]  IntegratorContinuousStateAttributes=''  IntegratorStateMustResolveToSignalObject=off  IntegratorRTWStateStorageClass=Auto  FilterContinuousStateAttributes=''  FilterStateMustResolveToSignalObject=off  FilterRTWStateStorageClass=Auto  ParallelPVariant=InternalParameters  IdealPVariant=Disabled  IVariant=InternalParameters  DVariant=InternalParameters  IntegratorVariant=Continuous  SatVariant=Disabled  AWVariant=Passthrough  PCopyVariant=Disabled  TRVariant=Disabled  FdbkBlocksVariant=Forward  IdealPFdbkVariant=Disabled  SatFdbkVariant=Disabled  DerivativeFilterVariant=ContFilter  NVariant=InternalParameters  NCopyVariant=Disabled  FilterICVariant=InternalICsFilter  IntegratorICVariant=InternalICs  ExternalResetVariant=Disabled  TRSumVariant=Passthrough  SumFdbkVariant=Disabled  SumVariant=Sum_PID
  Sensing Angle : Subsystem  RequirementInfo={} %GIDa_1f560d22_62cf_4135_99ab_9497af6cc4a9
      mask Display: disp('a')
  Shaft Free End : fl_lib/Mechanical/Rotational Elements/Rotational Free End  RequirementInfo={} %GIDa_96953efb_a144_4f53_8724_60d3e3d77e60  w_specify=off  w_priority=None  w=0 rad/s  w_nominal_specify=off  w_nominal_unit=rad/s  w_nominal_value=1
      settings: SourceProductBaseCode=SS
  Solver Configuration : nesl_utility/Solver Configuration  RequirementInfo={} %GIDa_a792cfaf_06d1_486e_83ad_c0232a19faa4  PhysicalDomain=network_engine_domain  SubClassName=solver  LeftPortType=input  RightPortType=generic  Tones=[]  Harmonics=[]  SimulateNoise=off  Profile=off  UseLocalSampling=off  EnableSwitchedLinearOptims=on  FrequencyDomain=off  UseCCode=off  RelTol=0.001  AbsTol=1e-06  MinStep=1e-09  ToWorkspace=off  RevertToSquareIcSolve=off  NumHomotopyIterations=100  PhasorMode=off  PhasorModeNumHarmonics=1  DoDC=off  ResidualTolerance=1e-9  UseLocalSolver=off  LocalSolverChoice=NE_BACKWARD_EULER_ADVANCER  LocalSolverSampleTime=.001  DoFixedCost=off  MaxNonlinIter=3  MaxModeIter=2  ComputeImpulses=off  ImpulseIterations=2  LinearAlgebra=auto  EquationFormulation=NE_TIME_EF  DelaysMemoryBudget=1024  AutomaticFiltering=on  FilteringTimeConstant=0.001  PartitionStorageMethod=AS_NEEDED  PartitionMemoryBudget=1024  PartitionMethod=FAST
      settings: SourceProductBaseCode=PW,SS
  Stepper Motor Driver : ee_lib/Electromechanical/Reluctance & Stepper/Stepper Motor Driver  RequirementInfo={} %GIDa_db1d4f75_853b_40bd_b8f2_1a7a605ced9e  step_or_av=ee.enum.electromech.simulationMode.stepping  step_rate_per_volt=10 Hz/V  Venable=2.5 V  Vreverse=2.5 V  supply_ports=ee.enum.supply_ports.hidesupply  Vm=5 V  Vsupply=10 V  half_stepping=ee.enum.electromech.steppingModeAveraged.fullStep  stepping_mode=ee.enum.electromech.steppingMode.microStep  numMicroSteps=4  Im=1.2 A
      settings: SourceProductBaseCode=PS  InternalSimscapePortConfiguration="{\"Bottom\":[],\"Left\":[{\"id\":\"ENA\",\"label\":\"ENA\",\"type\":\"foundation.electrical.electrical\"},{\"id\":\"REF\",\"label\":\"REF\",\"type\":\"foundation.electrical.electrical\"},{\"id\":\"REV\",\"label\":\"REV\",\"type\":\"foundation.electrical.electrical\"}],\"Right\":[{\"id\":\"pA\",\"label\":\"A+\",\"type\":\"foundation.electrical.electrical\"},{\"id\":\"nA\",\"label\":\"A-\",\"type\":\"foundation.electrical.electrical\"},{\"id\":\"pB\",\"label\":\"B+\",\"type\":\"foundation.electrical.electrical\"},{\"id\":\"nB\",\"label\":\"B-\",\"type\":\"foundation.electrical.electrical\"}],\"Top\":[]}"
  Stepper Motor4 : ee_lib/Electromechanical/Reluctance & Stepper/Stepper Motor  RequirementInfo={} %GIDa_ee01ad6b_6f68_4bfa_9f87_83074de87596  step_or_av=1  Ra=0.55 Ohm  La=0.0015 H  Km=0.19 N*m/A  Td=0 N*m  Rm=Inf Ohm  w_vec=[ 0 1000 3e+3 ] rpm  T_vec=[ 2 2 1 ] N*m  assert_if_slipping=0  J_total=1e-4 kg*m^2  max_step_rate=10 Hz  Step=1.8 deg  J=4.5e-05 kg*m^2  B=1e-02 N*m/(rad/s)  speed0=0 rpm  theta0=0 deg  alpha=[.00393, .00393] 1/K  Tmeas=25 degC  Tmeas2=125 degC  T_vec2=[1.7, 1.7, .85] N*m  half_stepping=ee.enum.electromech.steppingModeAveraged.fullStep  thermal_masses=[100, 100] J/K  initial_temperatures=[25, 25] degC  rotor_thermal_mass=50 J/K  rotor_initial_temperature=25 degC  Rm_percent_rotor=90
      settings: SourceProductBaseCode=PS  InternalSimscapePortConfiguration="{\"Bottom\":[],\"Left\":[{\"id\":\"pA\",\"label\":\"A+\",\"type\":\"foundation.electrical.electrical\"},{\"id\":\"nA\",\"label\":\"A-\",\"type\":\"foundation.electrical.electrical\"},{\"id\":\"pB\",\"label\":\"B+\",\"type\":\"foundation.electrical.electrical\"},{\"id\":\"nB\",\"label\":\"B-\",\"type\":\"foundation.electrical.electrical\"}],\"Right\":[{\"id\":\"R\",\"label\":\"R\",\"type\":\"foundation.mechanical.rotational.rotational\"},{\"id\":\"C\",\"label\":\"C\",\"type\":\"foundation.mechanical.rotational.rotational\"}],\"Top\":[]}"
  Sum : Sum  RequirementInfo={} %GIDa_4f32c526_f997_434a_b7b5_345181e5849e  Inputs=|+-
  theta4 : Outport  RequirementInfo={} %GIDa_2e71a2df_3566_489e_b203_4ca5dbd23898
  wires:
  PID Controller/1 -> Controller/1(Ref)
  Sensing Angle/1(theta) -> theta4/1, Delay One Step/1
  Sum/1 -> PID Controller/1
  In1/1 -> Sum/1
  Delay One Step/1 -> Sum/2
  connections:
  Stepper Motor4/RConn1 -- Shaft Free End/LConn1 -- Friction Stepper 4/LConn1 -- Sensing Angle/LConn1
  ERef B-/LConn1 -- Stepper Motor Driver/RConn4 -- Stepper Motor4/LConn4
  Controller/RConn3 -- Stepper Motor Driver/LConn3
  Mechanical Rotational Reference5/LConn1 -- Friction Stepper 4/RConn1
  Stepper Motor Driver/RConn3 -- Stepper Motor4/LConn3
  Stepper Motor Driver/RConn2 -- Stepper Motor4/LConn2 -- ERef A+/LConn1
  MRRef Motor/LConn1 -- Stepper Motor4/RConn2 -- Solver Configuration/RConn1
  Controller/RConn1 -- Stepper Motor Driver/LConn1
  Stepper Motor Driver/RConn1 -- Stepper Motor4/LConn1
  Controller/RConn2 -- Stepper Motor Driver/LConn2

== system Multilink_Robot_Arm_control/JOINT1/Controller ==
  Ref : Inport  RequirementInfo={} %GIDa_0d19dee1_68ae_440f_8960_81c4a15f8a51
  Speed : Subsystem  RequirementInfo={} %GIDa_8daf85ff_f308_4990_a8b7_144804c151b3  VariantControl=Speed
  PWM : PMIOPort  RequirementInfo={} %GIDa_089f4969_5eb6_4a6a_9b34_9f32067b556b  Side=Right
  0v : PMIOPort  RequirementInfo={} %GIDa_635e10e8_54c8_4ca7_ae0f_e7fe0bd13b5b  Port=2  Side=Right
  REV : PMIOPort  RequirementInfo={} %GIDa_a0b470d4_0b36_46cf_95d2_df5c8c74d0a8  Port=3  Side=Right

== system Multilink_Robot_Arm_control/JOINT1/Sensing Angle ==
  MRRef : fl_lib/Mechanical/Rotational Elements/Mechanical Rotational Reference  RequirementInfo={} %GIDa_03f12c93_a542_4ede_a5a9_f5b03d87814b
  Motion Sensor : fl_lib/Mechanical/Mechanical Sensors/Ideal Rotational Motion Sensor  RequirementInfo={} %GIDa_398a065d_7a12_4835_abbe_cbffd1c922f8  wrap_angle=simscape.enum.onoff.off  offset=0 rad
  deg : nesl_utility/PS-Simulink Converter  RequirementInfo={} %GIDa_5105d602_0145_4e54_ba41_c7bcfe77431f  PhysicalDomain=network_engine_domain  SubClassName=ps_output  LeftPortType=input  RightPortType=output  PseudoPeriodic=off  Frequencies=[]  Unit=deg  AffineConversion=off
      settings: SourceProductBaseCode=PW,SS
  R : PMIOPort  RequirementInfo={} %GIDa_14a917c4_1472_49e8_b6ab_859500374b16  Side=Left
  theta : Outport  RequirementInfo={} %GIDa_ad878903_c1f3_4f9a_acf9_e1efa9d2904d  VectorParamsAs1DForOutWhenUnconnected=off
  wires:
  deg/1 -> theta/1
  connections:
  MRRef/LConn1 -- Motion Sensor/RConn1
  Motion Sensor/RConn3 -- deg/LConn1
  R/RConn1 -- Motion Sensor/LConn1

== system Multilink_Robot_Arm_control/JOINT2/Controller ==
  Ref : Inport  RequirementInfo={} %GIDa_cb6c9f6b_785e_46d1_9148_7cdc04878a64
  Speed : Subsystem  RequirementInfo={} %GIDa_44bb5ea2_e961_45be_a774_60d9566b6c2f  VariantControl=Speed
  PWM : PMIOPort  RequirementInfo={} %GIDa_2628286a_c5a9_4811_8f97_e79ab35280c8  Side=Right
  0v : PMIOPort  RequirementInfo={} %GIDa_5f1d0535_2599_4231_8ec2_854e615db717  Port=2  Side=Right
  REV : PMIOPort  RequirementInfo={} %GIDa_5e490694_cbd4_4696_9679_56e6223c6a88  Port=3  Side=Right

== system Multilink_Robot_Arm_control/JOINT2/Sensing Angle ==
  MRRef : fl_lib/Mechanical/Rotational Elements/Mechanical Rotational Reference  RequirementInfo={} %GIDa_2c66323e_dd8c_411a_9618_3ff4be50bc4e
  Motion Sensor : fl_lib/Mechanical/Mechanical Sensors/Ideal Rotational Motion Sensor  RequirementInfo={} %GIDa_85a7bf56_acda_4d94_b121_46c48a1f0678  wrap_angle=simscape.enum.onoff.off  offset=0 rad
  deg : nesl_utility/PS-Simulink Converter  RequirementInfo={} %GIDa_99930954_b819_4ce6_b1a5_fbe6c23fd75d  PhysicalDomain=network_engine_domain  SubClassName=ps_output  LeftPortType=input  RightPortType=output  PseudoPeriodic=off  Frequencies=[]  Unit=deg  AffineConversion=off
      settings: SourceProductBaseCode=PW,SS
  R : PMIOPort  RequirementInfo={} %GIDa_e4c54a4c_f8c6_4d5b_a3ea_ce70f8e98a41  Side=Left
  theta : Outport  RequirementInfo={} %GIDa_b59844d5_c7cf_46ff_a462_0275027ccf99  VectorParamsAs1DForOutWhenUnconnected=off
  wires:
  deg/1 -> theta/1
  connections:
  R/RConn1 -- Motion Sensor/LConn1
  Motion Sensor/RConn3 -- deg/LConn1
  MRRef/LConn1 -- Motion Sensor/RConn1

== system Multilink_Robot_Arm_control/JOINT3/Controller ==
  Ref : Inport  RequirementInfo={} %GIDa_9a3e5d11_2b20_44a9_b4c0_95a186349056
  Speed : Subsystem  RequirementInfo={} %GIDa_c440c86e_a788_4fa3_b33a_9b00efb1a78d  VariantControl=Speed
  PWM : PMIOPort  RequirementInfo={} %GIDa_53a92660_41fc_4828_a7d8_b7cb2bb48210  Side=Right
  0v : PMIOPort  RequirementInfo={} %GIDa_48897f0d_9cd8_4e17_b442_0420c9b62e6d  Port=2  Side=Right
  REV : PMIOPort  RequirementInfo={} %GIDa_807f5c48_8bbf_435b_b570_9ece89da3ad4  Port=3  Side=Right

== system Multilink_Robot_Arm_control/JOINT3/Sensing Angle ==
  MRRef : fl_lib/Mechanical/Rotational Elements/Mechanical Rotational Reference  RequirementInfo={} %GIDa_1d4cf88c_0188_4f5c_a65c_9464b453cde6
  Motion Sensor : fl_lib/Mechanical/Mechanical Sensors/Ideal Rotational Motion Sensor  RequirementInfo={} %GIDa_41f5eec6_76e8_4c2c_b5ab_8c81acac81f4  wrap_angle=simscape.enum.onoff.off  offset=0 rad
  deg : nesl_utility/PS-Simulink Converter  RequirementInfo={} %GIDa_39924438_310a_4647_94eb_671062c09b17  PhysicalDomain=network_engine_domain  SubClassName=ps_output  LeftPortType=input  RightPortType=output  PseudoPeriodic=off  Frequencies=[]  Unit=deg  AffineConversion=off
      settings: SourceProductBaseCode=PW,SS
  R : PMIOPort  RequirementInfo={} %GIDa_1d575f6e_eb7b_4605_a6fe_9917c42d1bc0  Side=Left
  theta : Outport  RequirementInfo={} %GIDa_b1ab585c_62cc_49f8_9358_9b08fd7e9cea  VectorParamsAs1DForOutWhenUnconnected=off
  wires:
  deg/1 -> theta/1
  connections:
  MRRef/LConn1 -- Motion Sensor/RConn1
  Motion Sensor/RConn3 -- deg/LConn1
  R/RConn1 -- Motion Sensor/LConn1

== system Multilink_Robot_Arm_control/JOINT4/Controller ==
  Ref : Inport  RequirementInfo={} %GIDa_a275cd8a_89e7_4b0a_98ec_d8b1cf2e791b
  Speed : Subsystem  RequirementInfo={} %GIDa_5f6e643b_60e1_4273_9834_0381e9275c91  VariantControl=Speed
  PWM : PMIOPort  RequirementInfo={} %GIDa_11df51f2_12fc_4014_9781_5189ff805e44  Side=Right
  0v : PMIOPort  RequirementInfo={} %GIDa_7124c02e_8ff2_4c87_af86_9aa7907f54a5  Port=2  Side=Right
  REV : PMIOPort  RequirementInfo={} %GIDa_a12ba61c_3bf5_437b_8bac_6fff167062f3  Port=3  Side=Right

== system Multilink_Robot_Arm_control/JOINT4/Sensing Angle ==
  MRRef : fl_lib/Mechanical/Rotational Elements/Mechanical Rotational Reference  RequirementInfo={} %GIDa_3844893a_456b_429a_be9a_458198ebb5c7
  Motion Sensor : fl_lib/Mechanical/Mechanical Sensors/Ideal Rotational Motion Sensor  RequirementInfo={} %GIDa_d8bbf5ee_36a1_4f08_8f56_4eed7e10cda1  wrap_angle=simscape.enum.onoff.off  offset=0 rad
  deg : nesl_utility/PS-Simulink Converter  RequirementInfo={} %GIDa_71ea82c2_6a80_40ed_8fdf_9690a5e90436  PhysicalDomain=network_engine_domain  SubClassName=ps_output  LeftPortType=input  RightPortType=output  PseudoPeriodic=off  Frequencies=[]  Unit=deg  AffineConversion=off
      settings: SourceProductBaseCode=PW,SS
  R : PMIOPort  RequirementInfo={} %GIDa_fec82444_cdab_4430_b4e1_47c7f5967300  Side=Left
  theta : Outport  RequirementInfo={} %GIDa_5632ee97_0f41_41f2_98ca_e9b05f31130c  VectorParamsAs1DForOutWhenUnconnected=off
  wires:
  deg/1 -> theta/1
  connections:
  R/RConn1 -- Motion Sensor/LConn1
  Motion Sensor/RConn3 -- deg/LConn1
  MRRef/LConn1 -- Motion Sensor/RConn1

== system Multilink_Robot_Arm_control/JOINT1/Controller/Speed ==
  Ref : Inport  RequirementInfo={} %GIDa_d0ee7174_da2e_4a13_b8d1_69bd63c386f4
  ERef : fl_lib/Electrical/Electrical Elements/Electrical Reference  RequirementInfo={} %GIDa_d892a7c3_ff11_4861_b673_dad5452ce739
  Step Rate and Direction : Subsystem  RequirementInfo={} %GIDa_9ddd1ded_371e_438b_ae64_a8ff93102a04
  Voltage-Controlled Pulse Generator : Subsystem  RequirementInfo={} %GIDa_a04d5817_7cef_4d5c_9a76_06c0a45936c2
  PWM : PMIOPort  RequirementInfo={} %GIDa_6d9c0420_7d0f_4b7e_a43c_b651f1b52d5d  Side=Right
  0v : PMIOPort  RequirementInfo={} %GIDa_410845b1_f9e4_44cc_8010_55a4abd8c234  Port=2  Side=Right
  REV : PMIOPort  RequirementInfo={} %GIDa_c0e8388f_341a_4b9d_8a3e_88c0a827884f  Port=3  Side=Right
  wires:
  Ref/1 -> Step Rate and Direction/1(Reference)
  connections:
  Step Rate and Direction/RConn2 -- Voltage-Controlled Pulse Generator/LConn1
  Step Rate and Direction/RConn1 -- REV/RConn1
  ERef/LConn1 -- 0v/RConn1 -- Voltage-Controlled Pulse Generator/RConn2
  PWM/RConn1 -- Voltage-Controlled Pulse Generator/RConn1

== system Multilink_Robot_Arm_control/JOINT2/Controller/Speed ==
  Ref : Inport  RequirementInfo={} %GIDa_133d2fbd_c93e_4f77_b4ac_eab9d76c42d5
  ERef : fl_lib/Electrical/Electrical Elements/Electrical Reference  RequirementInfo={} %GIDa_7d76ed12_3202_4e07_9a81_a49e1b94768a
  Step Rate and Direction : Subsystem  RequirementInfo={} %GIDa_caaf0cf5_7010_465f_9918_d7533aa9d66e
  Voltage-Controlled Pulse Generator : Subsystem  RequirementInfo={} %GIDa_c6184c00_e7ae_4ed6_b023_dd2e423edd06
  PWM : PMIOPort  RequirementInfo={} %GIDa_212c39cb_5b57_476e_a698_4d1e9cdd5427  Side=Right
  0v : PMIOPort  RequirementInfo={} %GIDa_c3c92952_d7df_46f2_a6c1_61685cd34345  Port=2  Side=Right
  REV : PMIOPort  RequirementInfo={} %GIDa_dc8a3b62_1286_4359_8672_6bb9b44ae351  Port=3  Side=Right
  wires:
  Ref/1 -> Step Rate and Direction/1(Reference)
  connections:
  PWM/RConn1 -- Voltage-Controlled Pulse Generator/RConn1
  Voltage-Controlled Pulse Generator/RConn2 -- 0v/RConn1 -- ERef/LConn1
  Step Rate and Direction/RConn1 -- REV/RConn1
  Step Rate and Direction/RConn2 -- Voltage-Controlled Pulse Generator/LConn1

== system Multilink_Robot_Arm_control/JOINT3/Controller/Speed ==
  Ref : Inport  RequirementInfo={} %GIDa_816022ef_432a_4a79_90a7_2ae6cbd59fcd
  ERef : fl_lib/Electrical/Electrical Elements/Electrical Reference  RequirementInfo={} %GIDa_196008e7_2150_4d1c_9562_2b404e1eb384
  Step Rate and Direction : Subsystem  RequirementInfo={} %GIDa_3dc02a5d_9463_4040_a7f9_8c5ed42feb4d
  Voltage-Controlled Pulse Generator : Subsystem  RequirementInfo={} %GIDa_cda5a4f7_7bce_4a17_92d2_0249b497aa56
  PWM : PMIOPort  RequirementInfo={} %GIDa_ae6e6dfd_0883_41b5_a79f_f2a88b9bb8a5  Side=Right
  0v : PMIOPort  RequirementInfo={} %GIDa_84d0f212_669f_417f_b7e6_49da8841d292  Port=2  Side=Right
  REV : PMIOPort  RequirementInfo={} %GIDa_363b8ad7_587b_486d_9c01_9ecb04e88f52  Port=3  Side=Right
  wires:
  Ref/1 -> Step Rate and Direction/1(Reference)
  connections:
  Step Rate and Direction/RConn2 -- Voltage-Controlled Pulse Generator/LConn1
  Step Rate and Direction/RConn1 -- REV/RConn1
  ERef/LConn1 -- 0v/RConn1 -- Voltage-Controlled Pulse Generator/RConn2
  PWM/RConn1 -- Voltage-Controlled Pulse Generator/RConn1

== system Multilink_Robot_Arm_control/JOINT4/Controller/Speed ==
  Ref : Inport  RequirementInfo={} %GIDa_d717e889_664f_4dd2_8736_eb6c370576c8
  ERef : fl_lib/Electrical/Electrical Elements/Electrical Reference  RequirementInfo={} %GIDa_8f4f37d8_c331_48d0_9e36_178249331710
  Step Rate and Direction : Subsystem  RequirementInfo={} %GIDa_7f64dba6_34d7_4fd6_b7e6_8ef2aa4dbaeb
  Voltage-Controlled Pulse Generator : Subsystem  RequirementInfo={} %GIDa_cf4eb0bf_28be_416a_a242_a03039ffa540
  PWM : PMIOPort  RequirementInfo={} %GIDa_aef454f5_c686_4161_86a7_873aeed7fd4b  Side=Right
  0v : PMIOPort  RequirementInfo={} %GIDa_3be3be1f_d3f7_46ea_ae96_b67254762afc  Port=2  Side=Right
  REV : PMIOPort  RequirementInfo={} %GIDa_ffa23ca5_42c1_4813_9242_4a9203d3890b  Port=3  Side=Right
  wires:
  Ref/1 -> Step Rate and Direction/1(Reference)
  connections:
  PWM/RConn1 -- Voltage-Controlled Pulse Generator/RConn1
  Voltage-Controlled Pulse Generator/RConn2 -- 0v/RConn1 -- ERef/LConn1
  Step Rate and Direction/RConn1 -- REV/RConn1
  Step Rate and Direction/RConn2 -- Voltage-Controlled Pulse Generator/LConn1

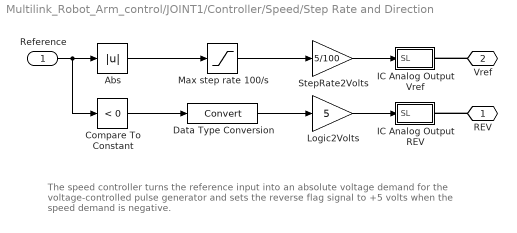
== system Multilink_Robot_Arm_control/JOINT1/Controller/Speed/Step Rate and Direction ==
  note: The speed controller turns the reference input into an absolute voltage demand for the
      | voltage-controlled pulse generator and sets the reverse flag signal to +5 volts when the
      | speed demand is negative.
  Reference : Inport  RequirementInfo={} %GIDa_a4d0a8f3_775c_42b8_9ce6_c57082dd7fd6
  Abs : Abs  RequirementInfo={} %GIDa_7613da56_6ee1_41bb_bf24_79eccb83e254
  Compare To Constant : simulink/Logic and Bit Operations/Compare To Constant  relop=<  const=0  OutDataTypeStr=uint8  ZeroCross=off
  Data Type Conversion : DataTypeConversion  RequirementInfo={} %GIDa_15417bf0_c7ec_4a8f_8ffd_c88ebbfd43ea
  IC Analog Output REV : Subsystem  RequirementInfo={} %GIDa_2381db1b_a9cd_4814_b69d_fad528507182
  IC Analog Output Vref : Subsystem  RequirementInfo={} %GIDa_7a2ed817_81c4_46ea_bee9_8975aad226ea
  Logic2Volts : Gain  RequirementInfo={} %GIDa_359c6216_a839_4c16_a394_d78c702d9162  Gain=5
  Max step rate 100/s : Saturate  RequirementInfo={} %GIDa_432da2a1_418c_4d16_83eb_56a19b9fecce  UpperLimit=100  LowerLimit=0
  StepRate2Volts : Gain  RequirementInfo={} %GIDa_aa390892_47b5_48bb_8fe1_8b1239142bf5  Gain=5/100
  REV : PMIOPort  RequirementInfo={} %GIDa_b21a2a82_f1de_4c93_a224_afadd27e55c2  Side=Right
  Vref : PMIOPort  RequirementInfo={} %GIDa_5a2899ae_9d44_4071_a42f_9f02a65277c8  Port=2  Side=Right
  wires:
  Logic2Volts/1 -> IC Analog Output REV/1(SL)
  Abs/1 -> Max step rate 100/s/1
  Reference/1 -> Abs/1, Compare To Constant/1
  Compare To Constant/1 -> Data Type Conversion/1
  Data Type Conversion/1 -> Logic2Volts/1
  Max step rate 100/s/1 -> StepRate2Volts/1
  StepRate2Volts/1 -> IC Analog Output Vref/1(SL)
  connections:
  Vref/RConn1 -- IC Analog Output Vref/RConn1
  REV/RConn1 -- IC Analog Output REV/RConn1
